simulink model "FMS"  (R2018b)
settings: configuration reference "FMS_config" (kept outside this file)
undefined symbols (not defined in the file): actuator_cmd, DiscIntNeverNeededParam, FMS_EXPORT, FMS_PARAM, mode, p_cmd, phi_cmd, psi_rate_cmd, q_cmd, r_cmd, reset, state, theta_cmd, throttle_cmd, timestamp, u_cmd, v_cmd, w_cmd
libraries: simulink x30, Rotation x2, Filter x1
(part 2 of 2)

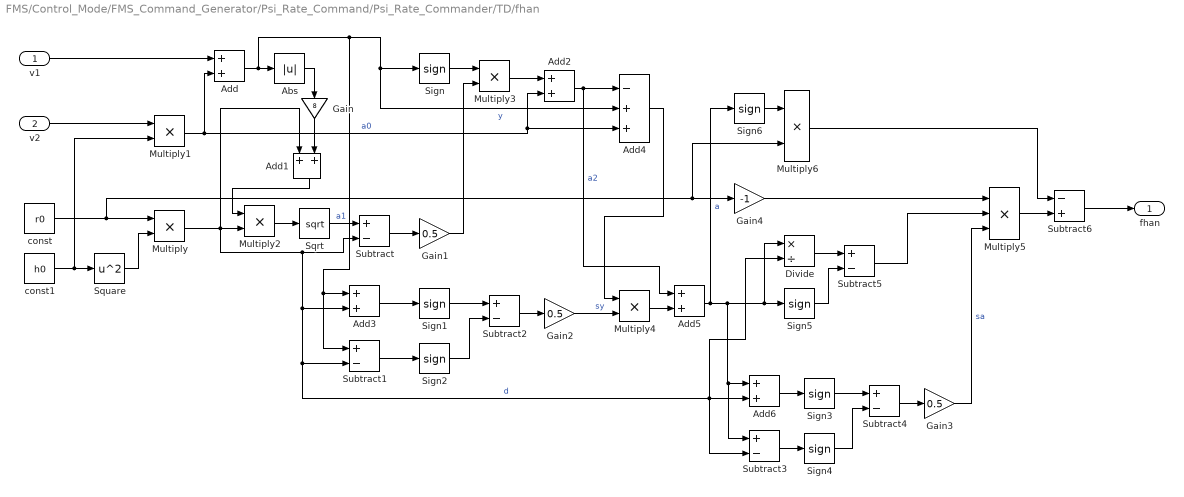
== system FMS/Control_Mode/FMS_Command_Generator/Psi_Rate_Command/Psi_Rate_Commander/TD/fhan  ==
  v1 : Inport
  v2 : Inport  Port=2
  Abs : Abs
  Add{,1..3,5..6} (6 alike) : Sum  OutDataTypeStr=Inherit: Same as first input
  Add4 : Sum  Inputs=-++
  Divide : Product  Inputs=*/
  Gain : Gain  Gain=8
  Gain1 : Gain  Gain=0.5  OutDataTypeStr=Inherit: Same as input
  Gain2 : Gain  Gain=0.5  OutDataTypeStr=Inherit: Same as input
  Gain3 : Gain  Gain=0.5  OutDataTypeStr=Inherit: Same as input
  Gain4 : Gain  Gain=-1  OutDataTypeStr=Inherit: Same as input
  Multiply{,1..3} (4 alike) : Product  OutDataTypeStr=Inherit: Same as first input
  Multiply4 : Product  OutDataTypeStr=single
  Multiply5 : Product  Inputs=3
  Multiply6 : Product  OutDataTypeStr=single
  Sign{,1..6} (7 alike) : Signum
  Sqrt : Sqrt  SaturateOnIntegerOverflow=on
  Square : Math  Operator=square  SaturateOnIntegerOverflow=on
  Subtract{,1..5} (6 alike) : Sum  Inputs=+-  OutDataTypeStr=Inherit: Same as first input
  Subtract6 : Sum  Inputs=-+  OutDataTypeStr=Inherit: Same as first input
  const : Constant  Value=r0  OutDataTypeStr=single
  const1 : Constant  Value=h0  OutDataTypeStr=single
  fhan : Outport
  wires:
  Sign1/1 -> Subtract2/1
  Multiply2/1 -> Sqrt/1
  Square/1 -> Multiply/2
  Gain1/1 -> Multiply3/2
  Multiply6/1 -> Subtract6/1
  Multiply/1 -> Multiply2/2, Add1/1, Add3/2, Subtract1/2, Add6/2, Subtract3/2, Divide/2, Subtract/2  "d"
  Add6/1 -> Sign3/1
  Sign3/1 -> Subtract4/1
  Sign6/1 -> Multiply6/1
  Multiply5/1 -> Subtract6/2
  Gain4/1 -> Multiply5/1
  Subtract4/1 -> Gain3/1
  Add2/1 -> Add5/1, Add4/1  "a2"
  Subtract2/1 -> Gain2/1
  Add/1 -> Abs/1, Sign/1, Add4/2, Add3/1, Subtract1/1  "y"
  Multiply1/1 -> Add/2, Add2/2, Add4/3  "a0"
  Add5/1 -> Add6/1, Subtract3/1, Divide/1, Sign5/1, Sign6/1  "a"
  const1/1 -> Square/1, Multiply1/2
  Multiply4/1 -> Add5/2
  Subtract5/1 -> Multiply5/2
  Add3/1 -> Sign1/1
  const/1 -> Multiply/1, Gain4/1, Multiply6/2
  Gain/1 -> Add1/2
  Multiply3/1 -> Add2/1
  Divide/1 -> Subtract5/1
  Subtract1/1 -> Sign2/1
  Add1/1 -> Multiply2/1
  Subtract3/1 -> Sign4/1
  Sqrt/1 -> Subtract/1  "a1"
  Sign5/1 -> Subtract5/2
  Add4/1 -> Multiply4/1
  Abs/1 -> Gain/1
  Sign4/1 -> Subtract4/2
  Sign2/1 -> Subtract2/2
  Subtract6/1 -> fhan/1
  Subtract/1 -> Gain1/1
  Gain3/1 -> Multiply5/3  "sa"
  v2/1 -> Multiply1/1
  Gain2/1 -> Multiply4/2  "sy"
  Sign/1 -> Multiply3/1
  v1/1 -> Add/1

== system FMS/Control_Mode/FMS_Command_Generator/Velocity_Command/Velocity_Commander/Motion_Speed/remap ==
  u : Inport
  Dead Zone : DeadZone  LowerValue=-th  UpperValue=th  SaturateOnIntegerOverflow=on
  Gain : Gain  Gain=1/(1-th)
  y : Outport
  wires:
  u/1 -> Dead Zone/1
  Dead Zone/1 -> Gain/1
  Gain/1 -> y/1

== system FMS/Control_Mode/FMS_Command_Generator/Velocity_Command/Velocity_Commander/Motion_Speed/remap1 ==
  u : Inport
  Dead Zone : DeadZone  LowerValue=-th  UpperValue=th  SaturateOnIntegerOverflow=on
  Gain : Gain  Gain=1/(1-th)
  y : Outport
  wires:
  Gain/1 -> y/1
  Dead Zone/1 -> Gain/1
  u/1 -> Dead Zone/1

== system FMS/Control_Mode/FMS_Command_Generator/Velocity_Command/Velocity_Commander/Motion_Speed/remap2 ==
  u : Inport
  Dead Zone : DeadZone  LowerValue=-th  UpperValue=th  SaturateOnIntegerOverflow=on
  Gain : Gain  Gain=1/(1-th)
  y : Outport
  wires:
  u/1 -> Dead Zone/1
  Dead Zone/1 -> Gain/1
  Gain/1 -> y/1

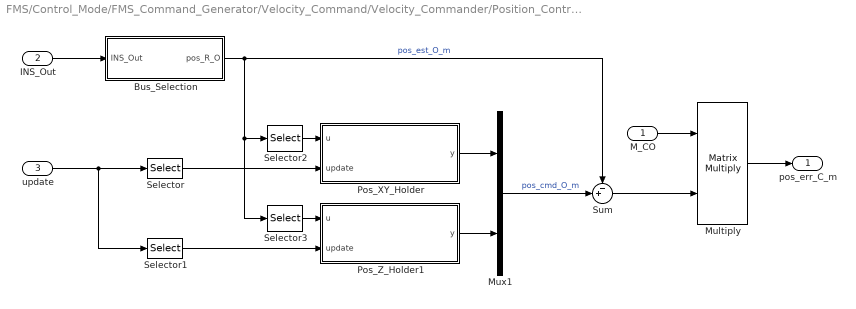
== system FMS/Control_Mode/FMS_Command_Generator/Velocity_Command/Velocity_Commander/Position_Control/Position_Error ==
  M_CO : Inport
  INS_Out : Inport  Port=2
  update : Inport  Port=3
  Bus_Selection : Subsystem
  Multiply : Product  Multiplication=Matrix(*)
  Mux1 : Mux  Inputs=2
  Pos_XY_Holder : Subsystem
  Pos_Z_Holder1 : Subsystem
  Selector : Selector  InputPortWidth=2  IndexOptions=Index vector (dialog)  Indices=1  OutputSizes=1
  Selector1 : Selector  InputPortWidth=2  IndexOptions=Index vector (dialog)  Indices=2  OutputSizes=1
  Selector2 : Selector  InputPortWidth=3  IndexOptions=Index vector (dialog)  Indices=[1 2]  OutputSizes=1
  Selector3 : Selector  InputPortWidth=3  IndexOptions=Index vector (dialog)  Indices=3  OutputSizes=1
  Sum : Sum  Inputs=-+|
  pos_err_C_m : Outport
  wires:
  Pos_XY_Holder/1(y) -> Mux1/1
  M_CO/1 -> Multiply/1
  Multiply/1 -> pos_err_C_m/1
  INS_Out/1 -> Bus_Selection/1(INS_Out)
  Bus_Selection/1(pos_R_O) -> Sum/1, Selector3/1, Selector2/1  "pos_est_O_m"
  update/1 -> Selector1/1, Selector/1
  Sum/1 -> Multiply/2
  Selector/1 -> Pos_XY_Holder/2(update)
  Selector1/1 -> Pos_Z_Holder1/2(update)
  Selector2/1 -> Pos_XY_Holder/1(u)
  Selector3/1 -> Pos_Z_Holder1/1(u)
  Mux1/1 -> Sum/2  "pos_cmd_O_m"
  Pos_Z_Holder1/1(y) -> Mux1/2

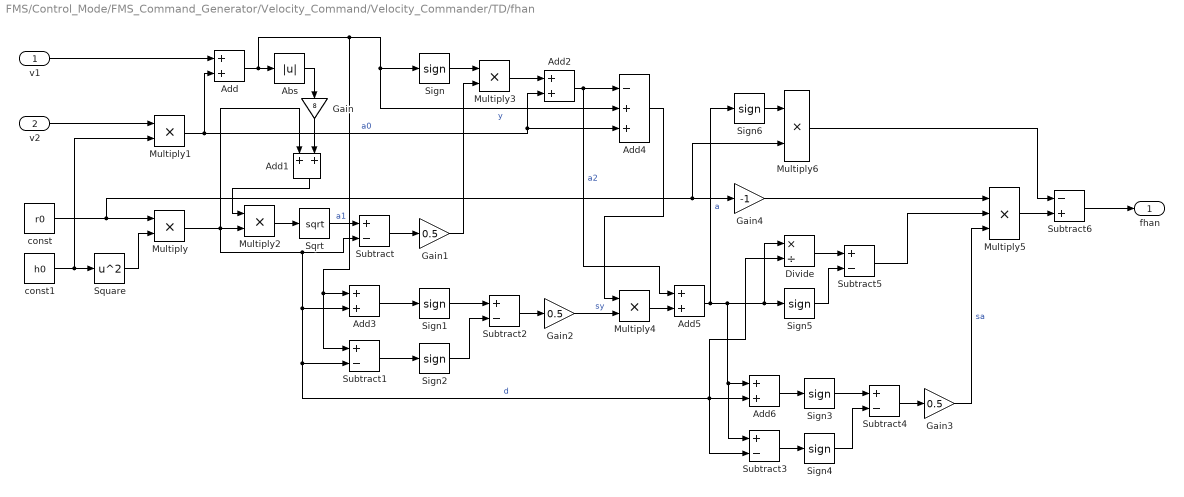
== system FMS/Control_Mode/FMS_Command_Generator/Velocity_Command/Velocity_Commander/TD/fhan  ==
  v1 : Inport
  v2 : Inport  Port=2
  Abs : Abs
  Add{,1..3,5..6} (6 alike) : Sum  OutDataTypeStr=Inherit: Same as first input
  Add4 : Sum  Inputs=-++
  Divide : Product  Inputs=*/
  Gain : Gain  Gain=8
  Gain1 : Gain  Gain=0.5  OutDataTypeStr=Inherit: Same as input
  Gain2 : Gain  Gain=0.5  OutDataTypeStr=Inherit: Same as input
  Gain3 : Gain  Gain=0.5  OutDataTypeStr=Inherit: Same as input
  Gain4 : Gain  Gain=-1  OutDataTypeStr=Inherit: Same as input
  Multiply{,1..3} (4 alike) : Product  OutDataTypeStr=Inherit: Same as first input
  Multiply4 : Product  OutDataTypeStr=single
  Multiply5 : Product  Inputs=3
  Multiply6 : Product  OutDataTypeStr=single
  Sign{,1..6} (7 alike) : Signum
  Sqrt : Sqrt  SaturateOnIntegerOverflow=on
  Square : Math  Operator=square  SaturateOnIntegerOverflow=on
  Subtract{,1..5} (6 alike) : Sum  Inputs=+-  OutDataTypeStr=Inherit: Same as first input
  Subtract6 : Sum  Inputs=-+  OutDataTypeStr=Inherit: Same as first input
  const : Constant  Value=r0  OutDataTypeStr=single
  const1 : Constant  Value=h0  OutDataTypeStr=single
  fhan : Outport
  wires:
  Sign1/1 -> Subtract2/1
  Multiply2/1 -> Sqrt/1
  Square/1 -> Multiply/2
  Gain1/1 -> Multiply3/2
  Multiply6/1 -> Subtract6/1
  Multiply/1 -> Multiply2/2, Add1/1, Add3/2, Subtract1/2, Add6/2, Subtract3/2, Divide/2, Subtract/2  "d"
  Add6/1 -> Sign3/1
  Sign3/1 -> Subtract4/1
  Sign6/1 -> Multiply6/1
  Multiply5/1 -> Subtract6/2
  Gain4/1 -> Multiply5/1
  Subtract4/1 -> Gain3/1
  Add2/1 -> Add5/1, Add4/1  "a2"
  Subtract2/1 -> Gain2/1
  Add/1 -> Abs/1, Sign/1, Add4/2, Add3/1, Subtract1/1  "y"
  Multiply1/1 -> Add/2, Add2/2, Add4/3  "a0"
  Add5/1 -> Add6/1, Subtract3/1, Divide/1, Sign5/1, Sign6/1  "a"
  const1/1 -> Square/1, Multiply1/2
  Multiply4/1 -> Add5/2
  Subtract5/1 -> Multiply5/2
  Add3/1 -> Sign1/1
  const/1 -> Multiply/1, Gain4/1, Multiply6/2
  Gain/1 -> Add1/2
  Multiply3/1 -> Add2/1
  Divide/1 -> Subtract5/1
  Subtract1/1 -> Sign2/1
  Add1/1 -> Multiply2/1
  Subtract3/1 -> Sign4/1
  Sqrt/1 -> Subtract/1  "a1"
  Sign5/1 -> Subtract5/2
  Add4/1 -> Multiply4/1
  Abs/1 -> Gain/1
  Sign4/1 -> Subtract4/2
  Sign2/1 -> Subtract2/2
  Subtract6/1 -> fhan/1
  Subtract/1 -> Gain1/1
  Gain3/1 -> Multiply5/3  "sa"
  v2/1 -> Multiply1/1
  Gain2/1 -> Multiply4/2  "sy"
  Sign/1 -> Multiply3/1
  v1/1 -> Add/1

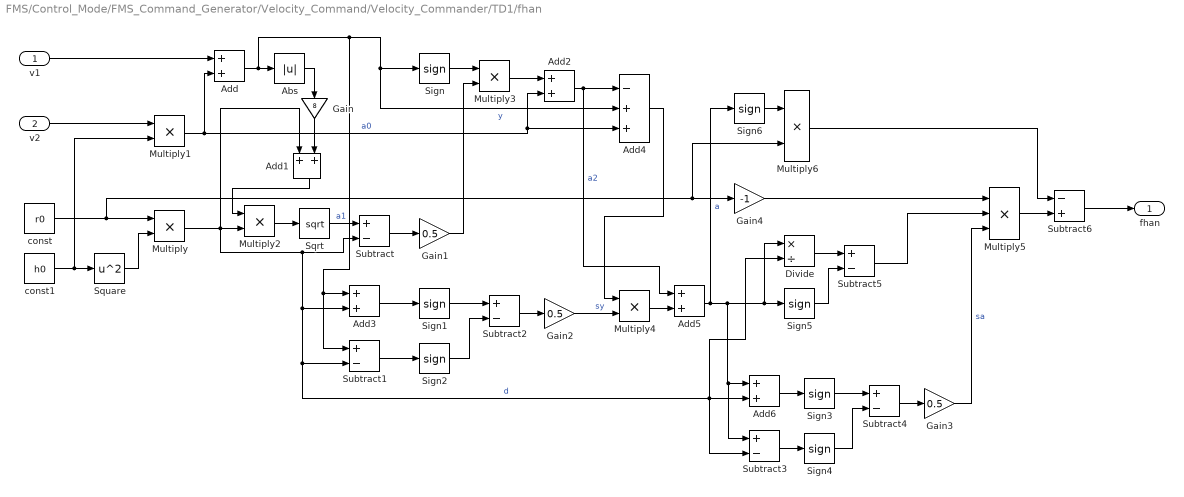
== system FMS/Control_Mode/FMS_Command_Generator/Velocity_Command/Velocity_Commander/TD1/fhan  ==
  v1 : Inport
  v2 : Inport  Port=2
  Abs : Abs
  Add{,1..3,5..6} (6 alike) : Sum  OutDataTypeStr=Inherit: Same as first input
  Add4 : Sum  Inputs=-++
  Divide : Product  Inputs=*/
  Gain : Gain  Gain=8
  Gain1 : Gain  Gain=0.5  OutDataTypeStr=Inherit: Same as input
  Gain2 : Gain  Gain=0.5  OutDataTypeStr=Inherit: Same as input
  Gain3 : Gain  Gain=0.5  OutDataTypeStr=Inherit: Same as input
  Gain4 : Gain  Gain=-1  OutDataTypeStr=Inherit: Same as input
  Multiply{,1..3} (4 alike) : Product  OutDataTypeStr=Inherit: Same as first input
  Multiply4 : Product  OutDataTypeStr=single
  Multiply5 : Product  Inputs=3
  Multiply6 : Product  OutDataTypeStr=single
  Sign{,1..6} (7 alike) : Signum
  Sqrt : Sqrt  SaturateOnIntegerOverflow=on
  Square : Math  Operator=square  SaturateOnIntegerOverflow=on
  Subtract{,1..5} (6 alike) : Sum  Inputs=+-  OutDataTypeStr=Inherit: Same as first input
  Subtract6 : Sum  Inputs=-+  OutDataTypeStr=Inherit: Same as first input
  const : Constant  Value=r0  OutDataTypeStr=single
  const1 : Constant  Value=h0  OutDataTypeStr=single
  fhan : Outport
  wires:
  Sign1/1 -> Subtract2/1
  Multiply2/1 -> Sqrt/1
  Square/1 -> Multiply/2
  Gain1/1 -> Multiply3/2
  Multiply6/1 -> Subtract6/1
  Multiply/1 -> Multiply2/2, Add1/1, Add3/2, Subtract1/2, Add6/2, Subtract3/2, Divide/2, Subtract/2  "d"
  Add6/1 -> Sign3/1
  Sign3/1 -> Subtract4/1
  Sign6/1 -> Multiply6/1
  Multiply5/1 -> Subtract6/2
  Gain4/1 -> Multiply5/1
  Subtract4/1 -> Gain3/1
  Add2/1 -> Add5/1, Add4/1  "a2"
  Subtract2/1 -> Gain2/1
  Add/1 -> Abs/1, Sign/1, Add4/2, Add3/1, Subtract1/1  "y"
  Multiply1/1 -> Add/2, Add2/2, Add4/3  "a0"
  Add5/1 -> Add6/1, Subtract3/1, Divide/1, Sign5/1, Sign6/1  "a"
  const1/1 -> Square/1, Multiply1/2
  Multiply4/1 -> Add5/2
  Subtract5/1 -> Multiply5/2
  Add3/1 -> Sign1/1
  const/1 -> Multiply/1, Gain4/1, Multiply6/2
  Gain/1 -> Add1/2
  Multiply3/1 -> Add2/1
  Divide/1 -> Subtract5/1
  Subtract1/1 -> Sign2/1
  Add1/1 -> Multiply2/1
  Subtract3/1 -> Sign4/1
  Sqrt/1 -> Subtract/1  "a1"
  Sign5/1 -> Subtract5/2
  Add4/1 -> Multiply4/1
  Abs/1 -> Gain/1
  Sign4/1 -> Subtract4/2
  Sign2/1 -> Subtract2/2
  Subtract6/1 -> fhan/1
  Subtract/1 -> Gain1/1
  Gain3/1 -> Multiply5/3  "sa"
  v2/1 -> Multiply1/1
  Gain2/1 -> Multiply4/2  "sy"
  Sign/1 -> Multiply3/1
  v1/1 -> Add/1

== system FMS/Control_Mode/FMS_Command_Generator/Psi_Rate_Command/Psi_Rate_Commander/Heading_Control/Heading_Error/Bus_Selection ==
  INS_Out : Inport
  Bus Selector2 : BusSelector  OutputSignals=psi
  psi_rad : Outport
  wires:
  INS_Out/1 -> Bus Selector2/1
  Bus Selector2/1 -> psi_rad/1  "<psi>"

== system FMS/Control_Mode/FMS_Command_Generator/Psi_Rate_Command/Psi_Rate_Commander/Heading_Control/Heading_Error/Psi_Holder ==
  u : Inport
  update : Inport  Port=2
  Delay : Delay  DelayLength=1  InitialConditionSource=Input port
      settings: InputPortMap=u0,p4
  Switch1 : Switch  Criteria=u2 > Threshold
  y : Outport
  wires:
  Switch1/1 -> y/1, Delay/1
  Delay/1 -> Switch1/3
  update/1 -> Switch1/2
  u/1 -> Delay/2, Switch1/1

== system FMS/Control_Mode/FMS_Command_Generator/Velocity_Command/Velocity_Commander/Position_Control/Position_Error/Bus_Selection ==
  INS_Out : Inport
  Bus Selector2 : BusSelector  OutputSignals=x_R,y_R,h_R
  Gain : Gain  Gain=-1
  Mux3 : Mux  Inputs=3
  pos_R_O : Outport
  wires:
  Mux3/1 -> pos_R_O/1
  Bus Selector2/1 -> Mux3/1  "<x_R>"
  Bus Selector2/2 -> Mux3/2  "<y_R>"
  INS_Out/1 -> Bus Selector2/1
  Bus Selector2/3 -> Gain/1  "<h_R>"
  Gain/1 -> Mux3/3

== system FMS/Control_Mode/FMS_Command_Generator/Velocity_Command/Velocity_Commander/Position_Control/Position_Error/Pos_XY_Holder ==
  u : Inport
  update : Inport  Port=2
  Delay : Delay  DelayLength=1  InitialConditionSource=Input port
      settings: InputPortMap=u0,p4
  Switch1 : Switch  Criteria=u2 > Threshold
  y : Outport
  wires:
  Switch1/1 -> y/1, Delay/1
  Delay/1 -> Switch1/3
  update/1 -> Switch1/2
  u/1 -> Delay/2, Switch1/1

== system FMS/Control_Mode/FMS_Command_Generator/Velocity_Command/Velocity_Commander/Position_Control/Position_Error/Pos_Z_Holder1 ==
  u : Inport
  update : Inport  Port=2
  Delay : Delay  DelayLength=1  InitialConditionSource=Input port
      settings: InputPortMap=u0,p4
  Switch1 : Switch  Criteria=u2 > Threshold
  y : Outport
  wires:
  Switch1/1 -> y/1, Delay/1
  Delay/1 -> Switch1/3
  update/1 -> Switch1/2
  u/1 -> Delay/2, Switch1/1

== stateflow chart FMS/Control_Mode/Control_Mode ==
  state Unknow
    entry:
    local_mode = 0;
  state Mission
    entry:
    local_mode = 1;
  state Position
    entry:
    local_mode = 2;
  state Altitude_Hold
    entry:
    local_mode = 3;
  state Manual
    entry:
    local_mode = 4;
  state Acro
    entry:
    local_mode = 5;
  (junction 126) -> Unknow
  Unknow -> (junction 130)
  (junction 115) -> (junction 126) [order 2]
  (junction 130) -> (junction 75)
  (junction 115) -> Mission [order 1] : [mode == 1]
  Mission -> (junction 73)
  (junction 73) -> (junction 75) [order 1] : [bitget(flag, 4) && bitget(flag, 6)]
  (junction 50) -> (junction 115) [order 2]
  (junction 73) -> Position [order 2]
  (junction 75) -> (junction 81)
  (junction 50) -> Position [order 1] : [mode == 2]
  Position -> (junction 79)
  (junction 79) -> (junction 81) [order 1] : [bitget(flag, 4) && bitget(flag, 7) && bitget(flag, 8)]
  (junction 53) -> (junction 50) [order 2]
  (junction 79) -> Altitude_Hold [order 2]
  (junction 81) -> (junction 90)
  (junction 53) -> Altitude_Hold [order 1] : [mode == 3]
  Altitude_Hold -> (junction 88)
  (junction 88) -> (junction 90) [order 1] : [bitget(flag, 8)]
  (junction 56) -> (junction 53) [order 2]
  (junction 88) -> Manual [order 2]
  (junction 90) -> (junction 98)
  (junction 56) -> Manual [order 1] : [mode == 4]
  Manual -> (junction 136)
  (junction 136) -> (junction 98) [order 1] : [bitget(flag, 3)]
  (junction 59) -> (junction 56) [order 2]
  (junction 136) -> Acro [order 2]
  (junction 98) -> (junction 103)
  (default) -> (junction 59)
  (junction 59) -> Acro [order 1] : [mode == 5]
  Acro -> (junction 103)
  (junction 108) -> (junction 59)
  (junction 103) -> (junction 106)
  (junction 106) -> (junction 108) : {control_mode = local_mode;}
  data: mode input; local_mode local uint32; flag input uint32; control_mode output

== stateflow chart FMS/Control_Mode/FMS_Command_Generator/Psi_Rate_Command/Motion_Check/Motion_State ==
  state Hold
    entry:
    state=2;
  state Move
    entry:
    state=0;
  state Brake
    entry:
    state=1;
  (default) -> Move
  Hold -> Move : [move_cmd==1]
  Move -> Brake : [move_cmd==0]
  Brake -> Move [order 2] : [move_cmd==1]
  Brake -> Hold [order 1] : [heading_rate<=0.1 || after(1, sec)]
  data: move_cmd input; heading_rate input; state output

== stateflow chart FMS/FMS_State/State_Management ==
  state Motor_Test
    entry:
    State = 1;
    during:
    PWM_Cmd = 1000 + uint16((stick_throttle+1)*500);
  state Disarm
    entry:
    State = 0;
    PWM_Cmd = 1000;
  state Arm
    entry:
    State = 2;
  state Standby
    entry:
    State = 1;
    PWM_Cmd = 1150;
  Disarm -> Motor_Test [order 1] : [test_motor_state == 1 && arm_event == 1]
  Motor_Test -> Disarm : [test_motor_state == 0 || arm_event == 1]
  (default) -> Disarm
  Arm -> Disarm [order 1] : [disarm_event == 1]
  Arm -> Disarm [order 2] : [force_disarm_event == 1]
  Disarm -> Standby [order 2] : [arm_event == 1]
  Standby -> Disarm [order 1] : after(30,sec)
  Standby -> Disarm [order 3] : [arm_event == 1 || force_disarm_event]
  Standby -> Arm [order 2] : [stick_throttle > -0.25]
  data: PWM_Cmd output uint16; State output; stick_throttle input; arm_event input; disarm_event input; force_disarm_event input; test_motor_state input

== stateflow chart FMS/Input_Process/Commander/Event_Commander/Arm_Disarm_Event/Arm_Event ==
  state Idle
    en:
    arm_event = 0;
  state arm_event
    en:
    arm_event = 1;
  state ready
  (default) -> Idle
  arm_event -> Idle
  Idle -> ready : [stick_throttle < -0.8 && stick_roll < -0.8 && stick_pitch < -0.8]
  ready -> arm_event : [abs(stick_roll) < 0.15 && abs(stick_pitch)<0.15]
  data: stick_roll input; stick_pitch input; stick_throttle input; arm_event output

== stateflow chart FMS/Control_Mode/FMS_Command_Generator/Velocity_Command/Motion_Check/Motion_State/Z_Motion_SM ==
  state Hold
    entry:
    state=2;
  state Move
    entry:
    state=0;
  state Brake
    entry:
    state=1;
  (default) -> Move
  Hold -> Move : [move_cmd==1]
  Move -> Brake : [move_cmd==0]
  Brake -> Move [order 2] : [move_cmd==1]
  Brake -> Hold [order 1] : [speed<=0.2 || after(1.5, sec)]
  data: move_cmd input; state output; speed input

== stateflow chart FMS/Input_Process/Commander/Event_Commander/Arm_Disarm_Event/Disarm_Event ==
  state Disarm
    en:
    disarm_event = 1;
  state Idle
    en:
    disarm_event = 0;
  state On_Ground
  (default) -> Idle
  Disarm -> Idle
  On_Ground -> Disarm [order 2] : [after(1.5, sec)]
  On_Ground -> Idle [order 1] : [on_ground == 0]
  Idle -> On_Ground : [on_ground == 1 && state == 2]
  data: on_ground input; disarm_event output; state input

== stateflow chart FMS/Control_Mode/FMS_Command_Generator/Velocity_Command/Motion_Check/Motion_State/XY_Motion_SM ==
  state Hold
    entry:
    state=2;
  state Move
    entry:
    state=0;
  state Brake
    entry:
    state=1;
  (default) -> Move
  Hold -> Move : [move_cmd==1]
  Move -> Brake : [move_cmd==0]
  Brake -> Move [order 2] : [move_cmd==1]
  Brake -> Hold [order 1] : [speed<=0.2 || after(2.5, sec)]
  data: move_cmd input; state output; speed input
